simulink library "SaliencyLib"  (Simulink 7.1)
undefined symbols (not defined in the file): isc, IScale, isr, oa
libraries: SaliencyLib x77
settings Model: Creator=bruce  LastModifiedBy=bruce

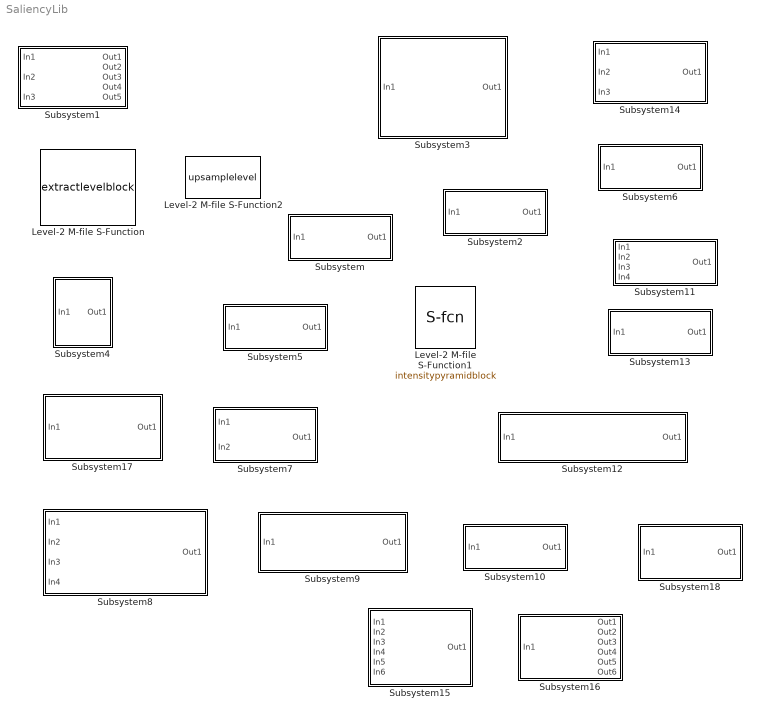
== system SaliencyLib ==
  Level-2 M-file S-Function : M-S-Function  FunctionName=extractlevelblock  Parameters=br,bc,pl,bo  mask(Extract Pyramid Level){br=332, bc=500, pl=2, bo=0}
      mask prompts: br "base rows:"; bc "base cols:"; pl "pyramid level:"; bo "base offset:"
      mask help:
      | Extracts one scale level from a multi-resolution pyramid
      | (that previously was packed into a matrix).
      mask Help:
      | For parameters are required.  Base rows and columns are the
      | dimensions of the level 0 image.  The pyramid level is the
      | resolution level that will be output. Base offset is normally
      | zero, but if the input pyramid was obtained by extracting
      | level n from a pyramid with level 0 dimensions given by the
      | base row and col parameter, then the base offset should be
      | set to n to give the correct input pyramid dimensions.
      mask Display: fprintf('EXTRACT\nLEVEL %s\n(%s x %s)', get_param(gcb, 'pl'),get_param(gcb,'br'),get_param(gcb,'bc'))
  Level-2 M-file S-Function1 : M-S-Function  FunctionName=intensitypyramidblock  Parameters=sr,sc,sl,bo  mask(Multi-Resolution Image Pyramid){sr=332, sc=500, sl=8, bo=0}
      mask prompts: sr "source rows:"; sc "source cols:"; sl "levels:"; bo "base offset:"
      mask help:
      | Constructs a multi-scale image pyramid from the input image
      | and outputs this pyramid packed into a 2-D matrix.
      mask Help:
      | Four parameters (sr,sc,sl,bo) are required.
      | 
      | sr and sc are the (nominal) row and column dimensions of the
      | input source image.
      | 
      | sl is the desired number of levels for the output pyramid.
      | 
      | bo is normally zero, but can be used to implicitly specify
      | the input image dimensions when the input is known to be
      | itself a level bo image from a pyramid derived from a base
      | image with dimensions sr by sc.
      mask Display: fprintf('PYRAMID\n(%s x %s)\n%s LEVEL', get_param(gcb,'sr'),get_param(gcb,'sc'),get_param(gcb,'sl'))
  Level-2 M-file S-Function2 : M-S-Function  FunctionName=upsamplelevel  Parameters=br,bc,fl,cl  mask(Upsample Image Pyramid Level){br=332, bc=500, fl=2, cl=5}
      mask prompts: br "base rows:"; bc "base cols:"; fl "fine level:"; cl "coarse level:"
      mask help:
      | Upsample a coarse resolution (higher) level image
      | to the resolution of a finer (lower) level image by simple
      | pixel replication.
      mask Help:
      | PARAMETERS:
      | base row, cols - level 0 image dimensions for the input pyramid.
      | fine level - the scale for the output image.
      | coarse level - the scale for the input image.
      mask Display: fprintf('UPSAMPLE\nLEVEL %s -> %s',get_param(gcb,'cl'),get_param(gcb,'fl'))
  Subsystem : Subsystem
      mask Type: Matrix Maximum
      mask Description: Outputs the value of the largest element in the input matrix.
      mask Display:
      | disp('MATRIX\nMAX')
      | port_label('input',1,'IMG')
      | port_label('output',1,'MAX')
  Subsystem1 : Subsystem  Tag=Color Map
      mask Type: Color Mapping
      mask Description:
      | Maps conventional RGB color component images to
      | intensity plus RGBY channels used by saliency algorithm.
      mask Display:
      | disp('COLOR\nMAPPING')
      | port_label('input',1,'r')
      | port_label('input',2','g')
      | port_label('input',3,'b')
      | port_label('output',1,'I')
      | port_label('output',2,'R')
      | port_label('output',3,'G')
      | port_label('output',4','B')
      | port_label('output',5,'Y')
  Subsystem10 : Subsystem  mask(Multi-Scale Color Opponent Saliency Channel){bRows=0, bCols=0}
      mask prompts: bRows "base rows:"; bCols "base cols:"
      mask help:
      | Outputs a bus containing color opponent saliency maps for
      | six different center-surround scale pairs.
      mask Display: fprintf('MULTI-SCALE\nCOLOR OPP\n(%s x %s)', get_param(gcb,'bRows'),get_param(gcb,'bCols'))
  Subsystem11 : Subsystem  mask(Color Based Saliency Channel){br=332, bc=500}
      mask prompts: br "base rows:"; bc "base cols:"
      mask help:
      | Outputs saliency map based on multi-scale double color
      | opponent center-surround differences in the input image.
      mask Display: fprintf('COLOR CHANNEL\n(%s x %s)',get_param(gcb,'br'),get_param(gcb,'bc'))
  Subsystem12 : Subsystem  mask(Single Orientation Saliency Channel){isr=332, isc=500, oa=0}
      mask prompts: isr "source rows:"; isc "source cols:"; oa "orientation angle:"
      mask help:
      | Outputs saliency map based on multi-scale center-surround
      | feature orientation differences for a single, parametrically
      | specified orientation.
      mask Display: fprintf('ORIENTED CHANNEL (%s DEG)\n(%s X %s)', get_param(gcb, 'oa'), get_param(gcb,'isr'),get_param(gcb,'isc'))
  Subsystem13 : Subsystem  mask(Multi-Orientation Based Saliency Channel){sr=0, sc=0}
      mask prompts: sr "source rows:"; sc "source cols:"
      mask help:
      | Outputs saliency map based on multi-scale, multi-orientation
      | center-surround feature orientation differences.
      mask Display: fprintf('MULTI-ORIENTED\nCHANNEL\n(%s x %s)',get_param(gcb,'sr'),get_param(gcb,'sc'))
  Subsystem14 : Subsystem  mask(Three Channel Saliency){inRows=332, inCols=500}
      mask prompts: inRows "input rows:"; inCols "input cols:"
      mask help:
      | Implements a three channel (intensity, orientation, color)
      | saliency map computaion based on the 1998 PAMI paper.
      mask Display:
      | fprintf('I-O-C CHANNEL\nSALIENCY\n(%s x %s)', get_param(gcb,'inRows'),get_param(gcb,'inCols'))
      | port_label('input',1,'r')
      | port_label('input',2,'g')
      | port_label('input',3,'b')
      | port_label('output',1,'SAL')
  Subsystem15 : Subsystem
      mask Type: Multi-Scale Image Bus Creator
      mask Description:
      | Provides a standardized means of assembling a multi-scale
      | collection of images into a bus.
      mask Display: disp('X-SCALE BUS\nCREATOR')
  Subsystem16 : Subsystem
      mask Type: Multi-Scale Image Bus Selector
      mask Description:
      | Provides a standardized connection to the bus created by
      | "X-SCALE BUS CREATOR" and un-packs bus components to separate
      | outputs.
      mask Display: disp('X-SCALE BUS\nSELECTOR')
  Subsystem17 : Subsystem  mask(Cross-Scale Summation){brxs=322, bcxs=500, L1off=0, L2off=0}
      mask prompts: brxs "base rows:"; bcxs "base cols:"; L1off "level one offset:"; L2off "level two offset:"
      mask help:
      | Output is the sum of six input center-surround absolute
      | difference maps at three different scales. Scales are
      | combined by downsampling.
      mask Display: fprintf('X-SCALE\nCOMBINE\n(%s x %s)\n%d-%d',get_param(gcb,'brxs'),get_param(gcb,'bcxs'),L1off,L2off)
  Subsystem18 : Subsystem  AncestorBlock=SaliencyLib/Subsystem12/Subsystem2  mask(Orientation Image Pyramid){sr=isr, sc=isc, pl=8, a=oa}
      mask prompts: sr "source rows:"; sc "source cols:"; pl "levels"; a "angle:"
      mask help:
      | Outputs a multi-scale pyramid obtained by applying a Gabor
      | kernel (with a parametrically specified orientation) to the
      | input image. The output pyramid is packed into a 2-D array.
      mask Display:
      | fprintf('ORIENT\nPYRAMID\n%s',get_param(gcb,'a'))
      | port_label('output',1,'PYR')
      | port_label('input',1,'IMG')
  Subsystem2 : Subsystem
      mask Type: Intensity Pyramid (DEPRECATED)
      mask Description:
      | Constructs a multi-scale image pyramid from the input matrix.
      | All of the pyramid levels are packed into a 2-D matrix.
      mask Display:
      | disp('INTENSITY\nPYRAMID')
      | port_label('output',1,'PYR')
      | port_label('input',1,'IMG')
  Subsystem3 : Subsystem  mask(Cross Level Difference){isr=0, isc=0}
      mask prompts: isr "input rows"; isc "input cols"
      mask help:
      | Computes absolute difference of scale 2 and 5 levels of an
      | image pyramid (upsampling the scale 5 image).
      mask Display:
      | port_label('input',1,'PYR')
      | port_label('output',1,'IMG')
      | fprintf('X-LEVEL DIFF\n(%d X %d)', isr, isc)
  Subsystem4 : Subsystem
      mask Type: Average of Local Maxima
      mask Description: Outputs average value of local maxima in the input image.
      mask Display: disp('AVG\nLOCAL\nMAX')
  Subsystem5 : Subsystem
      mask Type: Local Inhibition (Saliency Normalization)
      mask Description:
      | Scales input image based on difference of the global maximum
      | and the average of the local maxima.
      mask Display: disp('LOCAL\nINHIBIT')
  Subsystem6 : Subsystem  mask(Intensity Based Saliency Channel){isr=256, isc=256}
      mask prompts: isr "source rows:"; isc "source cols:"
      mask help:
      | Outputs a saliency map based on mulit-scale center-surround
      | intensity differences in the input image.
      mask Display: fprintf('INTENSITY CHANNEL\n(%s X %s)', get_param(gcb,'isr'),get_param(gcb,'isc'))
  Subsystem7 : Subsystem  mask(Color Opponent Pair Differences){br=332, bc=500, cl=2, sl=5}
      mask prompts: br "base rows:"; bc "base cols:"; cl "center level:"; sl "surround level:"
      mask help:
      | Computes multi-scale center-surround differences
      | for color opponent pairs.
      mask Display: fprintf('COLOR OPP\n(%s x %s)\n(%s -> %s)', get_param(gcb, 'br'), get_param(gcb, 'bc'), get_param(gcb, 'cl'), get_param(gcb, 'sl'))
  Subsystem8 : Subsystem  mask(Multi-Resolution Color Pyramid){br=332, bc=500}
      mask prompts: br "base rows:"; bc "base cols:"
      mask help:
      | Outputs a bus containing multi-resolution pyramids for each
      | of the four input color channel images.
      mask Display:
      | fprintf('COLOR PYRAMID\n(%s x %s)', get_param(gcb, 'br'), get_param(gcb, 'bc'))
      | port_label('input', 1, 'R')
      | port_label('input', 2', 'G')
      | port_label('input', 3, 'B')
      | port_label('input', 4, 'Y')
      | port_label('output', 1, 'CLRPY')
  Subsystem9 : Subsystem  mask(Single Resolution Color Opponent Saliency Channel){br=332, bc=500, cl=2, sl=5}
      mask prompts: br "base rows:"; bc "base cols:"; cl "center level:"; sl "surround level:"
      mask help:
      | Outputs a color opponent based saliency map for a
      | parametrically specified pair of center and surround
      | resolution scales.
      mask Display:
      | fprintf('CLR LEVEL\n(%s x %s)\n%s -> %s',get_param(gcb, 'br'),get_param(gcb, 'bc'),get_param(gcb,'cl'),get_param(gcb,'sl'))
      | port_label('input', 1, 'CLRPY')
      | port_label('output', 1, 'CPAIR')

== system SaliencyLib/Subsystem ==
  In1 : Inport  OutDataType=sfix(16)  OutScaling=2^0
  MATLAB Fcn : MATLABFcn  MATLABFcn=max(u(:))  Output1D=off
  Out1 : Outport  OutDataType=sfix(16)  OutScaling=2^0
  wires:
  MATLAB Fcn/1 -> Out1/1
  In1/1 -> MATLAB Fcn/1

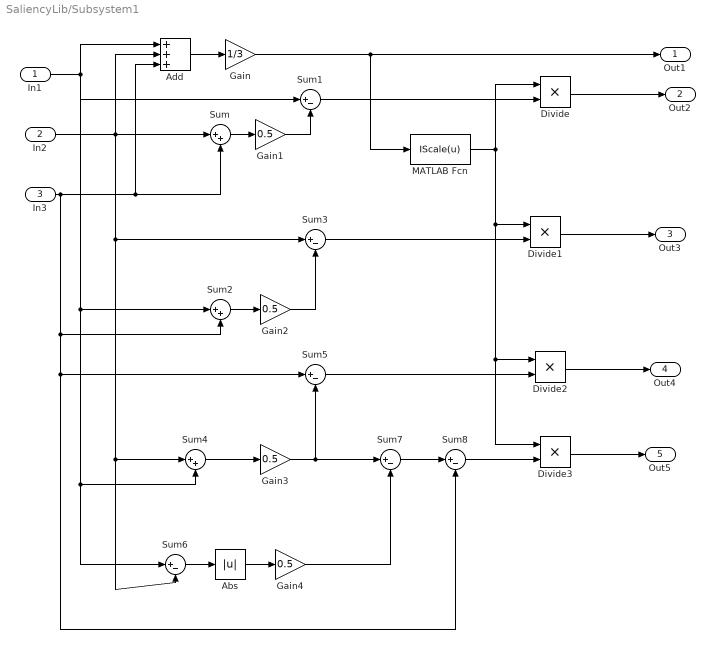
== system SaliencyLib/Subsystem1 ==
  In1 : Inport  OutDataType=sfix(16)  OutScaling=2^0
  In2 : Inport  Port=2  OutDataType=sfix(16)  OutScaling=2^0
  In3 : Inport  Port=3  OutDataType=sfix(16)  OutScaling=2^0
  Abs : Abs  OutDataType=sfix(16)  OutScaling=2^0
  Add : Sum  Inputs=+++  OutDataType=sfix(16)  OutScaling=2^-10
  Divide{,1..3} (4 alike) : Product  Inputs=**  OutDataType=sfix(16)  OutScaling=2^-10
  Gain : Gain  Gain=1/3  ParameterDataType=sfix(16)  ParameterScaling=2^0  OutDataType=sfix(16)  OutScaling=2^0
  Gain{1..4} (4 alike) : Gain  Gain=0.5  ParameterDataType=sfix(16)  ParameterScaling=2^0  OutDataType=sfix(16)  OutScaling=2^0
  MATLAB Fcn : MATLABFcn  MATLABFcn=IScale(u)  Output1D=off
  Sum : Sum  Inputs=|++  OutDataType=sfix(16)  OutScaling=2^0
  Sum{1,3,5..8} (6 alike) : Sum  Inputs=|+-  OutDataType=sfix(16)  OutScaling=2^0
  Sum2 : Sum  Inputs=|++  OutDataType=sfix(16)  OutScaling=2^0
  Sum4 : Sum  Inputs=|++  OutDataType=sfix(16)  OutScaling=2^0
  Out1 : Outport  OutDataType=sfix(16)  OutScaling=2^0
  Out2 : Outport  Port=2  OutDataType=sfix(16)  OutScaling=2^0
  Out3 : Outport  Port=3  OutDataType=sfix(16)  OutScaling=2^0
  Out4 : Outport  Port=4  OutDataType=sfix(16)  OutScaling=2^0
  Out5 : Outport  Port=5  OutDataType=sfix(16)  OutScaling=2^0
  wires:
  MATLAB Fcn/1 -> Divide3/1, Divide2/1, Divide1/1, Divide/1
  Divide3/1 -> Out5/1
  Sum8/1 -> Divide3/2
  Sum7/1 -> Sum8/1
  Gain4/1 -> Sum7/2
  Abs/1 -> Gain4/1
  Sum6/1 -> Abs/1
  Divide2/1 -> Out4/1
  Divide1/1 -> Out3/1
  Sum5/1 -> Divide2/2
  Sum3/1 -> Divide1/2
  Divide/1 -> Out2/1
  Sum1/1 -> Divide/2
  Sum4/1 -> Gain3/1
  Gain3/1 -> Sum7/1, Sum5/2
  Gain2/1 -> Sum3/2
  Sum2/1 -> Gain2/1
  Gain1/1 -> Sum1/2
  Sum/1 -> Gain1/1
  Add/1 -> Gain/1
  Gain/1 -> MATLAB Fcn/1, Out1/1
  In3/1 -> Sum8/2, Sum5/1, Sum2/2, Sum/2, Add/3
  In2/1 -> Sum6/2, Sum4/1, Sum3/1, Sum/1, Add/2
  In1/1 -> Sum6/1, Sum4/2, Sum2/1, Sum1/1, Add/1

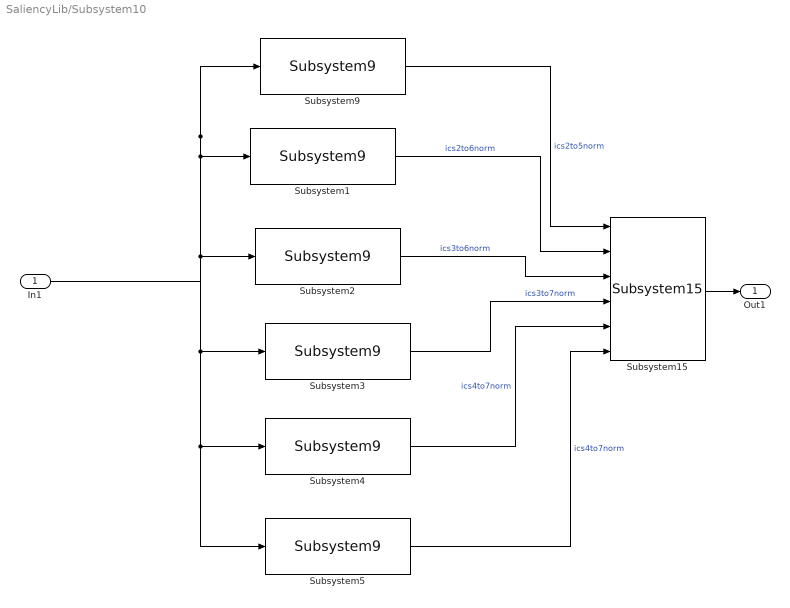
== system SaliencyLib/Subsystem10 ==
  In1 : Inport  OutDataType=sfix(16)  OutScaling=2^0
  Subsystem1 : SaliencyLib/Subsystem9  SystemSampleTime=-1  br=bRows  bc=bCols  cl=2  sl=6
  Subsystem15 : SaliencyLib/Subsystem15  SystemSampleTime=-1
  Subsystem2 : SaliencyLib/Subsystem9  SystemSampleTime=-1  br=bRows  bc=bCols  cl=3  sl=6
  Subsystem3 : SaliencyLib/Subsystem9  SystemSampleTime=-1  br=bRows  bc=bCols  cl=3  sl=7
  Subsystem4 : SaliencyLib/Subsystem9  SystemSampleTime=-1  br=bRows  bc=bCols  cl=4  sl=7
  Subsystem5 : SaliencyLib/Subsystem9  SystemSampleTime=-1  br=bRows  bc=bCols  cl=4  sl=8
  Subsystem9 : SaliencyLib/Subsystem9  SystemSampleTime=-1  br=bRows  bc=bCols  cl=2  sl=5
  Out1 : Outport  OutDataType=sfix(16)  OutScaling=2^0
  wires:
  In1/1 -> Subsystem9/1, Subsystem1/1, Subsystem2/1, Subsystem3/1, Subsystem4/1, Subsystem5/1
  Subsystem9/1 -> Subsystem15/1  "ics2to5norm"
  Subsystem1/1 -> Subsystem15/2  "ics2to6norm"
  Subsystem2/1 -> Subsystem15/3  "ics3to6norm"
  Subsystem3/1 -> Subsystem15/4  "ics3to7norm"
  Subsystem4/1 -> Subsystem15/5  "ics4to7norm"
  Subsystem5/1 -> Subsystem15/6  "ics4to7norm"
  Subsystem15/1 -> Out1/1

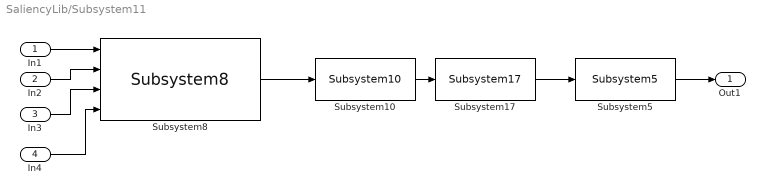
== system SaliencyLib/Subsystem11 ==
  In1 : Inport  OutDataType=sfix(16)  OutScaling=2^0
  In2 : Inport  Port=2  OutDataType=sfix(16)  OutScaling=2^0
  In3 : Inport  Port=3  OutDataType=sfix(16)  OutScaling=2^0
  In4 : Inport  Port=4  OutDataType=sfix(16)  OutScaling=2^0
  Subsystem10 : SaliencyLib/Subsystem10  SystemSampleTime=-1  bRows=br  bCols=bc
  Subsystem17 : SaliencyLib/Subsystem17  SystemSampleTime=-1  brxs=br  bcxs=bc  L1off=2  L2off=3
      link override Level-2 M-file S-Function6: bo=L2off
  Subsystem5 : SaliencyLib/Subsystem5  SystemSampleTime=-1
  Subsystem8 : SaliencyLib/Subsystem8  SystemSampleTime=-1  br=br  bc=bc
  Out1 : Outport  OutDataType=sfix(16)  OutScaling=2^0
  wires:
  In1/1 -> Subsystem8/1
  Subsystem8/1 -> Subsystem10/1
  Subsystem10/1 -> Subsystem17/1
  Subsystem17/1 -> Subsystem5/1
  Subsystem5/1 -> Out1/1
  In2/1 -> Subsystem8/2
  In3/1 -> Subsystem8/3
  In4/1 -> Subsystem8/4

== system SaliencyLib/Subsystem12 ==
  In1 : Inport  OutDataType=sfix(16)  OutScaling=2^0
  Subsystem12 : Subsystem
      mask Display: disp('NORMALIZE')
  Subsystem17 : SaliencyLib/Subsystem17  SystemSampleTime=-1  brxs=isr  bcxs=isc  L1off=2  L2off=3
  Subsystem2 : Subsystem  mask{sr=isr, sc=isc, pl=8, a=oa}
      mask prompts: sr "source rows:"; sc "source cols:"; pl "levels"; a "angle:"
      mask Display:
      | fprintf('ORIENT\nPYRAMID\n%s',get_param(gcb,'a'))
      | port_label('output',1,'PYR')
      | port_label('input',1,'IMG')
  Subsystem5 : SaliencyLib/Subsystem5  SystemSampleTime=-1
  Subsystem7 : Subsystem
      mask Display:
      | disp('C/S\nCOMBINE')
      | port_label('input',1,'PYR')
      | port_label('output',1,'I-BUS')
  Out1 : Outport  OutDataType=sfix(16)  OutScaling=2^0
  wires:
  In1/1 -> Subsystem2/1(In1)
  Subsystem2/1(Out1) -> Subsystem7/1(In1)
  Subsystem7/1(Out1) -> Subsystem12/1(In1)
  Subsystem17/1 -> Subsystem5/1
  Subsystem5/1 -> Out1/1
  Subsystem12/1(Out1) -> Subsystem17/1

== system SaliencyLib/Subsystem13 ==
  In1 : Inport  OutDataType=sfix(16)  OutScaling=2^0
  Add : Sum  Inputs=++++  OutDataType=sfix(16)  OutScaling=2^-10
  Subsystem1 : SaliencyLib/Subsystem12  SystemSampleTime=-1  isr=332  isc=500  oa=45
  Subsystem12 : SaliencyLib/Subsystem12  SystemSampleTime=-1  isr=332  isc=500  oa=0
  Subsystem2 : SaliencyLib/Subsystem12  SystemSampleTime=-1  isr=332  isc=500  oa=90
  Subsystem3 : SaliencyLib/Subsystem12  SystemSampleTime=-1  isr=332  isc=500  oa=135
  Subsystem5 : SaliencyLib/Subsystem5  SystemSampleTime=-1
  Out1 : Outport  OutDataType=sfix(16)  OutScaling=2^0
  wires:
  In1/1 -> Subsystem12/1, Subsystem1/1, Subsystem2/1, Subsystem3/1
  Subsystem12/1 -> Add/1
  Subsystem1/1 -> Add/2
  Subsystem2/1 -> Add/3
  Subsystem3/1 -> Add/4
  Add/1 -> Subsystem5/1
  Subsystem5/1 -> Out1/1

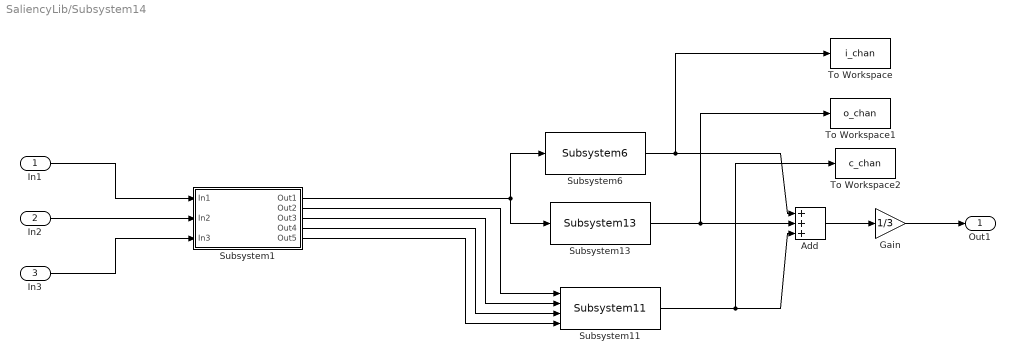
== system SaliencyLib/Subsystem14 ==
  In1 : Inport  OutDataType=sfix(16)  OutScaling=2^0
  In2 : Inport  Port=2  OutDataType=sfix(16)  OutScaling=2^0
  In3 : Inport  Port=3  OutDataType=sfix(16)  OutScaling=2^0
  Add : Sum  Inputs=+++  OutDataType=sfix(16)  OutScaling=2^-10
  Gain : Gain  Gain=1/3  ParameterDataType=sfix(16)  ParameterScaling=2^0  OutDataType=sfix(16)  OutScaling=2^0
  Subsystem1 : Subsystem
      mask Display:
      | disp('COLOR\nMAPPING')
      | port_label('input',1,'r')
      | port_label('input',2','g')
      | port_label('input',3,'b')
      | port_label('output',1,'I')
      | port_label('output',2,'R')
      | port_label('output',3,'G')
      | port_label('output',4','B')
      | port_label('output',5,'Y')
  Subsystem11 : SaliencyLib/Subsystem11  SystemSampleTime=-1  br=inRows  bc=inCols
  Subsystem13 : SaliencyLib/Subsystem13  SystemSampleTime=-1  sr=inRows  sc=inCols
  Subsystem6 : SaliencyLib/Subsystem6  SystemSampleTime=-1  isr=inRows  isc=inCols
      link override Subsystem17/Level-2 M-file S-Function: br=83  bc=125
      link override Subsystem17/Level-2 M-file S-Function1: sr=83  sc=125
      link override Subsystem17/Level-2 M-file S-Function2: sr=83  sc=125
      link override Subsystem17/Level-2 M-file S-Function3: sr=42  sc=63
      link override Subsystem17/Level-2 M-file S-Function4: sr=42  sc=63
      link override Subsystem17/Level-2 M-file S-Function5: br=83  bc=125
      link override Subsystem17/Level-2 M-file S-Function6: br=42  bc=63
      link override Subsystem17/Level-2 M-file S-Function7: br=42  bc=63
  To Workspace : ToWorkspace  VariableName=i_chan  SampleTime=-1  SaveFormat=Structure
  To Workspace1 : ToWorkspace  VariableName=o_chan  SampleTime=-1  SaveFormat=Structure
  To Workspace2 : ToWorkspace  VariableName=c_chan  SampleTime=-1  SaveFormat=Structure
  Out1 : Outport  OutDataType=sfix(16)  OutScaling=2^0
  wires:
  Add/1 -> Gain/1
  Gain/1 -> Out1/1
  Subsystem13/1 -> To Workspace1/1, Add/2
  Subsystem6/1 -> To Workspace/1, Add/1
  Subsystem11/1 -> To Workspace2/1, Add/3
  Subsystem1/5(Out5) -> Subsystem11/4
  Subsystem1/4(Out4) -> Subsystem11/3
  Subsystem1/3(Out3) -> Subsystem11/2
  Subsystem1/2(Out2) -> Subsystem11/1
  In3/1 -> Subsystem1/3(In3)
  In2/1 -> Subsystem1/2(In2)
  Subsystem1/1(Out1) -> Subsystem13/1, Subsystem6/1
  In1/1 -> Subsystem1/1(In1)

== system SaliencyLib/Subsystem15 ==
  In1 : Inport  OutDataType=sfix(16)  OutScaling=2^0
  In2 : Inport  Port=2  OutDataType=sfix(16)  OutScaling=2^0
  In3 : Inport  Port=3  OutDataType=sfix(16)  OutScaling=2^0
  In4 : Inport  Port=4  OutDataType=sfix(16)  OutScaling=2^0
  In5 : Inport  Port=5  OutDataType=sfix(16)  OutScaling=2^0
  In6 : Inport  Port=6  OutDataType=sfix(16)  OutScaling=2^0
  Bus Creator : BusCreator  Inputs='ics2to5norm','ics2to6norm','ics3to6norm','ics3to7norm','ics4to7norm','ics4to8norm'
  Out1 : Outport  OutDataType=sfix(16)  OutScaling=2^0
  wires:
  Bus Creator/1 -> Out1/1
  In1/1 -> Bus Creator/1  "ics2to5norm"
  In2/1 -> Bus Creator/2  "ics2to6norm"
  In3/1 -> Bus Creator/3  "ics3to6norm"
  In4/1 -> Bus Creator/4  "ics3to7norm"
  In5/1 -> Bus Creator/5  "ics4to7norm"
  In6/1 -> Bus Creator/6  "ics4to8norm"

== system SaliencyLib/Subsystem16 ==
  In1 : Inport  OutDataType=sfix(16)  OutScaling=2^0
  Bus Selector : BusSelector  OutputSignals=ics2to5norm,ics2to6norm,ics3to6norm,ics3to7norm,ics4to7norm,ics4to8norm
  Out1 : Outport  OutDataType=sfix(16)  OutScaling=2^0
  Out2 : Outport  Port=2  OutDataType=sfix(16)  OutScaling=2^0
  Out3 : Outport  Port=3  OutDataType=sfix(16)  OutScaling=2^0
  Out4 : Outport  Port=4  OutDataType=sfix(16)  OutScaling=2^0
  Out5 : Outport  Port=5  OutDataType=sfix(16)  OutScaling=2^0
  Out6 : Outport  Port=6  OutDataType=sfix(16)  OutScaling=2^0
  wires:
  In1/1 -> Bus Selector/1
  Bus Selector/1 -> Out1/1
  Bus Selector/2 -> Out2/1
  Bus Selector/3 -> Out3/1
  Bus Selector/4 -> Out4/1
  Bus Selector/5 -> Out5/1
  Bus Selector/6 -> Out6/1

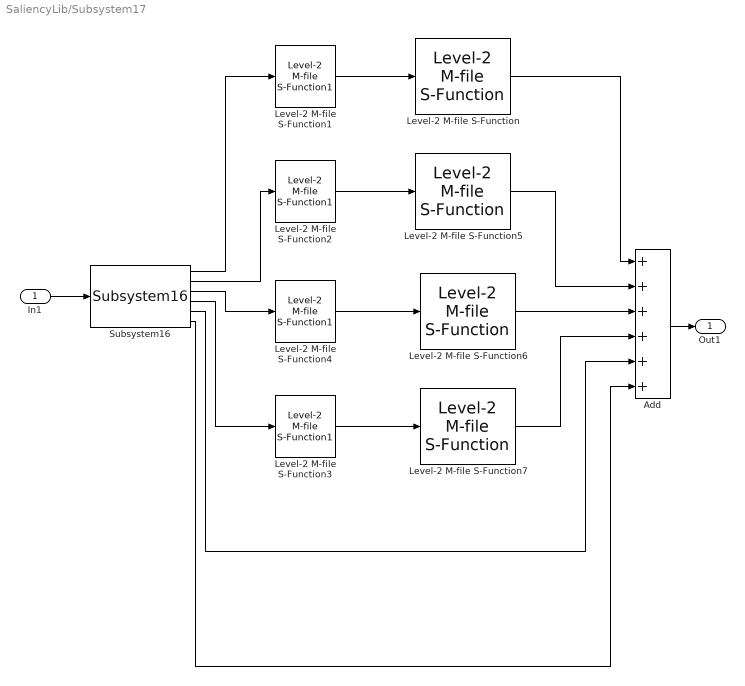
== system SaliencyLib/Subsystem17 ==
  In1 : Inport  OutDataType=sfix(16)  OutScaling=2^0
  Add : Sum  Inputs=++++++  OutDataType=sfix(16)  OutScaling=2^-10
  Level-2 M-file S-Function : SaliencyLib/Level-2 M-file S-Function  br=brxs  bc=bcxs  pl=2  bo=L1off
  Level-2 M-file S-Function1 : SaliencyLib/Level-2 M-file S-Function1  sr=brxs  sc=bcxs  sl=2  bo=0
  Level-2 M-file S-Function2 : SaliencyLib/Level-2 M-file S-Function1  sr=brxs  sc=bcxs  sl=2  bo=0
  Level-2 M-file S-Function3 : SaliencyLib/Level-2 M-file S-Function1  sr=brxs  sc=bcxs  sl=1  bo=0
  Level-2 M-file S-Function4 : SaliencyLib/Level-2 M-file S-Function1  sr=brxs  sc=bcxs  sl=1  bo=0
  Level-2 M-file S-Function5 : SaliencyLib/Level-2 M-file S-Function  br=brxs  bc=bcxs  pl=2  bo=L1off
  Level-2 M-file S-Function6 : SaliencyLib/Level-2 M-file S-Function  br=brxs  bc=bcxs  pl=1  bo=L2off
  Level-2 M-file S-Function7 : SaliencyLib/Level-2 M-file S-Function  br=brxs  bc=bcxs  pl=1  bo=L2off
  Subsystem16 : SaliencyLib/Subsystem16  SystemSampleTime=-1
  Out1 : Outport  OutDataType=sfix(16)  OutScaling=2^0
  wires:
  Add/1 -> Out1/1
  Level-2 M-file S-Function7/1 -> Add/4
  Level-2 M-file S-Function6/1 -> Add/3
  Level-2 M-file S-Function5/1 -> Add/2
  Level-2 M-file S-Function/1 -> Add/1
  Level-2 M-file S-Function3/1 -> Level-2 M-file S-Function7/1
  Level-2 M-file S-Function4/1 -> Level-2 M-file S-Function6/1
  Level-2 M-file S-Function2/1 -> Level-2 M-file S-Function5/1
  Level-2 M-file S-Function1/1 -> Level-2 M-file S-Function/1
  In1/1 -> Subsystem16/1
  Subsystem16/1 -> Level-2 M-file S-Function1/1
  Subsystem16/2 -> Level-2 M-file S-Function2/1
  Subsystem16/3 -> Level-2 M-file S-Function4/1
  Subsystem16/4 -> Level-2 M-file S-Function3/1
  Subsystem16/5 -> Add/5
  Subsystem16/6 -> Add/6

== system SaliencyLib/Subsystem18 ==
  In1 : Inport  OutDataType=sfix(16)  OutScaling=2^0
  Level-2 M-file S-Function : M-S-Function  FunctionName=orientationpyramidblock  Parameters=sr,sc,pl,a
  Out1 : Outport  OutDataType=sfix(16)  OutScaling=2^0
  wires:
  Level-2 M-file S-Function/1 -> Out1/1
  In1/1 -> Level-2 M-file S-Function/1

== system SaliencyLib/Subsystem2 ==
  In1 : Inport  OutDataType=sfix(16)  OutScaling=2^0
  MATLAB Fcn : MATLABFcn  MATLABFcn=IntensityPyramid  OutputDimensions=[499 500]  Output1D=off
  Out1 : Outport  OutDataType=sfix(16)  OutScaling=2^0
  wires:
  MATLAB Fcn/1 -> Out1/1
  In1/1 -> MATLAB Fcn/1

== system SaliencyLib/Subsystem3 ==
  In1 : Inport
  Abs : Abs  OutDataType=sfix(16)  OutScaling=2^0
  Level-2 M-file S-Function : SaliencyLib/Level-2 M-file S-Function  br=isr  bc=isc  pl=2  bo=0
  Level-2 M-file S-Function1 : SaliencyLib/Level-2 M-file S-Function  br=isr  bc=isc  pl=5  bo=0
  Level-2 M-file S-Function2 : SaliencyLib/Level-2 M-file S-Function2  br=isr  bc=isc  fl=2  cl=5
  Subtract : Sum  Inputs=+-  OutDataType=sfix(16)  OutScaling=2^-10
  Out1 : Outport
  wires:
  Level-2 M-file S-Function1/1 -> Level-2 M-file S-Function2/1
  Level-2 M-file S-Function2/1 -> Subtract/2
  Subtract/1 -> Abs/1
  Level-2 M-file S-Function/1 -> Subtract/1
  In1/1 -> Level-2 M-file S-Function1/1, Level-2 M-file S-Function/1
  Abs/1 -> Out1/1

== system SaliencyLib/Subsystem4 ==
  In1 : Inport  OutDataType=sfix(16)  OutScaling=2^0
  MATLAB Fcn1 : MATLABFcn  MATLABFcn=LocalMaxStats  Output1D=off
  Out1 : Outport  OutDataType=sfix(16)  OutScaling=2^0
  wires:
  In1/1 -> MATLAB Fcn1/1
  MATLAB Fcn1/1 -> Out1/1

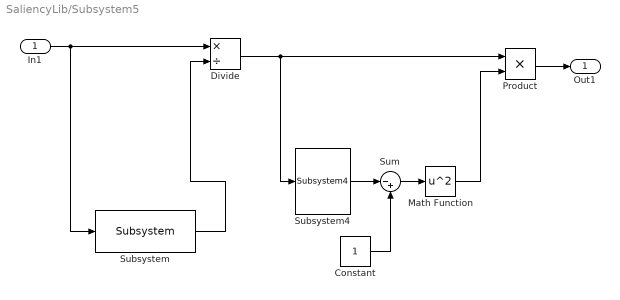
== system SaliencyLib/Subsystem5 ==
  In1 : Inport  OutDataType=sfix(16)  OutScaling=2^0
  Constant : Constant  OutDataType=sfix(16)  OutScaling=2^0
  Divide : Product  Inputs=*/  OutDataType=sfix(16)  OutScaling=2^-10
  Math Function : Math  Operator=square  OutDataType=sfix(16)  OutScaling=2^0  SaturateOnIntegerOverflow=on
  Product : Product  OutDataType=sfix(16)  OutScaling=2^0  RndMeth=Zero
  Subsystem : SaliencyLib/Subsystem  SystemSampleTime=-1
  Subsystem4 : SaliencyLib/Subsystem4  SystemSampleTime=-1
  Sum : Sum  Inputs=|-+  OutDataType=sfix(16)  OutScaling=2^0
  Out1 : Outport  OutDataType=sfix(16)  OutScaling=2^0
  wires:
  In1/1 -> Subsystem/1, Divide/1
  Subsystem/1 -> Divide/2
  Divide/1 -> Subsystem4/1, Product/1
  Constant/1 -> Sum/2
  Subsystem4/1 -> Sum/1
  Sum/1 -> Math Function/1
  Math Function/1 -> Product/2
  Product/1 -> Out1/1

== system SaliencyLib/Subsystem6 ==
  In1 : Inport  OutDataType=sfix(16)  OutScaling=2^0
  Level-2 M-file S-Function1 : SaliencyLib/Level-2 M-file S-Function1  sr=isr  sc=isc  sl=8  bo=0
  Subsystem12 : Subsystem
      mask Display: disp('NORMALIZE')
  Subsystem17 : SaliencyLib/Subsystem17  SystemSampleTime=-1  brxs=322  bcxs=500  L1off=0  L2off=0
  Subsystem5 : SaliencyLib/Subsystem5  SystemSampleTime=-1
  Subsystem7 : Subsystem
      mask Display:
      | disp('C/S\nCOMBINE')
      | port_label('input',1,'PYR')
      | port_label('output',1,'I-BUS')
  Out1 : Outport  OutDataType=sfix(16)  OutScaling=2^0
  wires:
  In1/1 -> Level-2 M-file S-Function1/1
  Level-2 M-file S-Function1/1 -> Subsystem7/1(In1)
  Subsystem7/1(Out1) -> Subsystem12/1(In1)
  Subsystem17/1 -> Subsystem5/1
  Subsystem5/1 -> Out1/1
  Subsystem12/1(Out1) -> Subsystem17/1

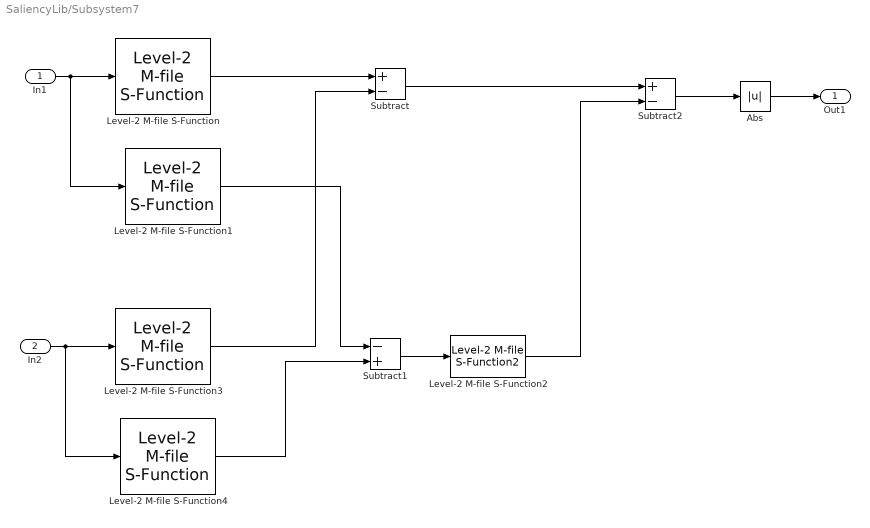
== system SaliencyLib/Subsystem7 ==
  In1 : Inport
  In2 : Inport  Port=2
  Abs : Abs  OutDataType=sfix(16)  OutScaling=2^0
  Level-2 M-file S-Function : SaliencyLib/Level-2 M-file S-Function  br=br  bc=bc  pl=cl  bo=0
  Level-2 M-file S-Function1 : SaliencyLib/Level-2 M-file S-Function  br=br  bc=bc  pl=sl  bo=0
  Level-2 M-file S-Function2 : SaliencyLib/Level-2 M-file S-Function2  br=br  bc=bc  fl=cl  cl=sl
  Level-2 M-file S-Function3 : SaliencyLib/Level-2 M-file S-Function  br=br  bc=bc  pl=cl  bo=0
  Level-2 M-file S-Function4 : SaliencyLib/Level-2 M-file S-Function  br=br  bc=bc  pl=sl  bo=0
  Subtract : Sum  Inputs=+-  OutDataType=sfix(16)  OutScaling=2^-10
  Subtract1 : Sum  Inputs=-+  OutDataType=sfix(16)  OutScaling=2^-10
  Subtract2 : Sum  Inputs=+-  OutDataType=sfix(16)  OutScaling=2^-10
  Out1 : Outport
  wires:
  Level-2 M-file S-Function/1 -> Subtract/1
  In1/1 -> Level-2 M-file S-Function1/1, Level-2 M-file S-Function/1
  Subtract1/1 -> Level-2 M-file S-Function2/1
  Level-2 M-file S-Function3/1 -> Subtract/2
  In2/1 -> Level-2 M-file S-Function3/1, Level-2 M-file S-Function4/1
  Level-2 M-file S-Function1/1 -> Subtract1/1
  Level-2 M-file S-Function4/1 -> Subtract1/2
  Abs/1 -> Out1/1
  Subtract/1 -> Subtract2/1
  Level-2 M-file S-Function2/1 -> Subtract2/2
  Subtract2/1 -> Abs/1

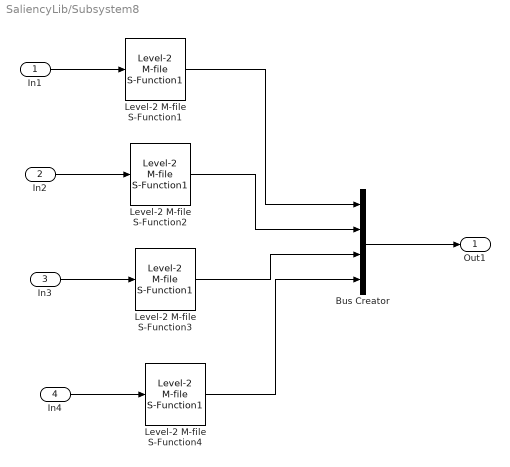
== system SaliencyLib/Subsystem8 ==
  In1 : Inport  OutDataType=sfix(16)  OutScaling=2^0
  In2 : Inport  Port=2  OutDataType=sfix(16)  OutScaling=2^0
  In3 : Inport  Port=3  OutDataType=sfix(16)  OutScaling=2^0
  In4 : Inport  Port=4  OutDataType=sfix(16)  OutScaling=2^0
  Bus Creator : BusCreator
  Level-2 M-file S-Function{1..4} (4 alike) : SaliencyLib/Level-2 M-file S-Function1  sr=332  sc=500  sl=8  bo=0
  Out1 : Outport  OutDataType=sfix(16)  OutScaling=2^0
  wires:
  In4/1 -> Level-2 M-file S-Function4/1
  In3/1 -> Level-2 M-file S-Function3/1
  In2/1 -> Level-2 M-file S-Function2/1
  In1/1 -> Level-2 M-file S-Function1/1
  Level-2 M-file S-Function1/1 -> Bus Creator/1
  Level-2 M-file S-Function2/1 -> Bus Creator/2
  Level-2 M-file S-Function3/1 -> Bus Creator/3
  Level-2 M-file S-Function4/1 -> Bus Creator/4
  Bus Creator/1 -> Out1/1

== system SaliencyLib/Subsystem9 ==
  In1 : Inport  OutDataType=sfix(16)  OutScaling=2^0
  Bus Selector : BusSelector  OutputSignals=signal1,signal2,signal3,signal4
  Subsystem1 : SaliencyLib/Subsystem7  SystemSampleTime=-1  br=br  bc=bc  cl=cl  sl=sl
  Subsystem2 : SaliencyLib/Subsystem5  SystemSampleTime=-1
  Subsystem5 : SaliencyLib/Subsystem5  SystemSampleTime=-1
  Subsystem7 : SaliencyLib/Subsystem7  SystemSampleTime=-1  br=br  bc=bc  cl=cl  sl=sl
  Sum : Sum  Inputs=|++  OutDataType=sfix(16)  OutScaling=2^0
  Out1 : Outport  OutDataType=sfix(16)  OutScaling=2^0
  wires:
  Sum/1 -> Out1/1
  In1/1 -> Bus Selector/1
  Bus Selector/1 -> Subsystem7/1  "<signal1>"
  Bus Selector/2 -> Subsystem7/2  "<signal2>"
  Bus Selector/3 -> Subsystem1/1  "<signal3>"
  Bus Selector/4 -> Subsystem1/2  "<signal4>"
  Subsystem7/1 -> Subsystem5/1
  Subsystem1/1 -> Subsystem2/1
  Subsystem5/1 -> Sum/1
  Subsystem2/1 -> Sum/2

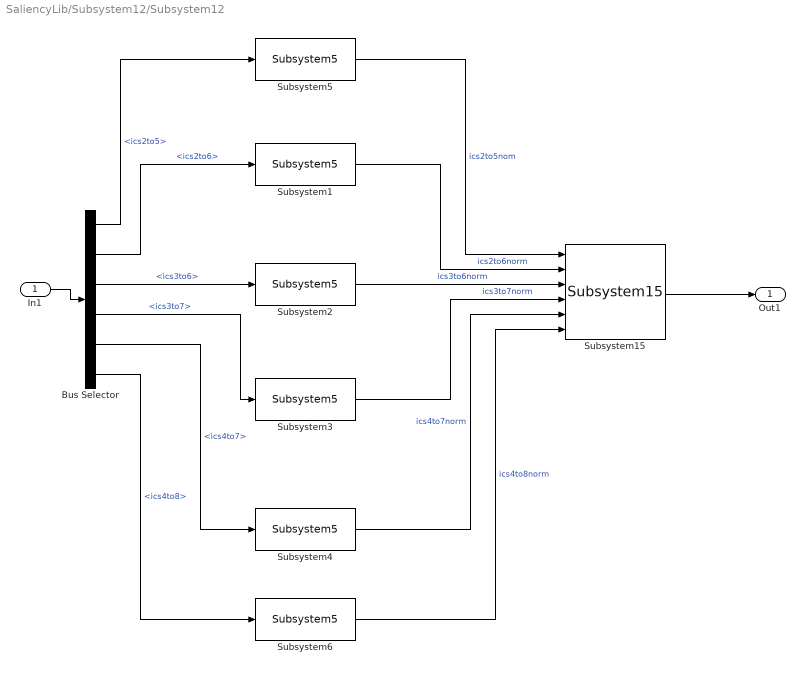
== system SaliencyLib/Subsystem12/Subsystem12 ==
  In1 : Inport  OutDataType=sfix(16)  OutScaling=2^0
  Bus Selector : BusSelector  OutputSignals=ics2to5,ics2to6,ics3to6,ics3to7,ics4to7,ics4to8
  Subsystem{1..6} (6 alike) : SaliencyLib/Subsystem5  SystemSampleTime=-1
  Subsystem15 : SaliencyLib/Subsystem15  SystemSampleTime=-1
  Out1 : Outport  OutDataType=sfix(16)  OutScaling=2^0
  wires:
  In1/1 -> Bus Selector/1
  Bus Selector/1 -> Subsystem5/1  "<ics2to5>"
  Bus Selector/2 -> Subsystem1/1  "<ics2to6>"
  Bus Selector/3 -> Subsystem2/1  "<ics3to6>"
  Bus Selector/4 -> Subsystem3/1  "<ics3to7>"
  Bus Selector/5 -> Subsystem4/1  "<ics4to7>"
  Bus Selector/6 -> Subsystem6/1  "<ics4to8>"
  Subsystem5/1 -> Subsystem15/1  "ics2to5nom"
  Subsystem1/1 -> Subsystem15/2  "ics2to6norm"
  Subsystem2/1 -> Subsystem15/3  "ics3to6norm"
  Subsystem3/1 -> Subsystem15/4  "ics3to7norm"
  Subsystem4/1 -> Subsystem15/5  "ics4to7norm"
  Subsystem6/1 -> Subsystem15/6  "ics4to8norm"
  Subsystem15/1 -> Out1/1

== system SaliencyLib/Subsystem12/Subsystem2 ==
  In1 : Inport  OutDataType=sfix(16)  OutScaling=2^0
  Level-2 M-file S-Function : M-S-Function  FunctionName=orientationpyramidblock  Parameters=sr,sc,pl,a
  Out1 : Outport  OutDataType=sfix(16)  OutScaling=2^0
  wires:
  In1/1 -> Level-2 M-file S-Function/1
  Level-2 M-file S-Function/1 -> Out1/1

== system SaliencyLib/Subsystem12/Subsystem7 ==
  In1 : Inport  OutDataType=sfix(16)  OutScaling=2^0
  Bus Creator : BusCreator  Inputs=6
  Subsystem1 : SaliencyLib/Subsystem3  SystemSampleTime=-1
      link override Level-2 M-file S-Function1: Parameters=332,500,6  pl=6
      link override Level-2 M-file S-Function2: cl=6
  Subsystem2 : SaliencyLib/Subsystem3  SystemSampleTime=-1
      link override Level-2 M-file S-Function: Parameters=332,500,3  pl=3
      link override Level-2 M-file S-Function1: Parameters=332,500,6  pl=6
      link override Level-2 M-file S-Function2: fl=3  cl=6
  Subsystem3 : SaliencyLib/Subsystem3  SystemSampleTime=-1
      link override Level-2 M-file S-Function: br=isr  bc=isc
      link override Level-2 M-file S-Function1: Parameters=332,500,5
  Subsystem4 : SaliencyLib/Subsystem3  SystemSampleTime=-1
      link override Level-2 M-file S-Function: Parameters=332,500,3  pl=3
      link override Level-2 M-file S-Function1: Parameters=332,500,7  pl=7
      link override Level-2 M-file S-Function2: fl=3  cl=7
  Subsystem5 : SaliencyLib/Subsystem3  SystemSampleTime=-1
      link override Level-2 M-file S-Function: Parameters=332,500,4  pl=4
      link override Level-2 M-file S-Function1: Parameters=332,500,7  pl=7
      link override Level-2 M-file S-Function2: fl=4  cl=7
  Subsystem6 : SaliencyLib/Subsystem3  SystemSampleTime=-1
      link override Level-2 M-file S-Function: Parameters=332,500,4  pl=4
      link override Level-2 M-file S-Function1: Parameters=332,500,8  pl=8
      link override Level-2 M-file S-Function2: fl=4  cl=8
  Out1 : Outport  OutDataType=sfix(16)  OutScaling=2^0
  wires:
  In1/1 -> Subsystem2/1, Subsystem4/1, Subsystem5/1, Subsystem6/1, Subsystem1/1, Subsystem3/1
  Subsystem1/1 -> Bus Creator/2  "ics2to6"
  Subsystem2/1 -> Bus Creator/3  "ics3to6"
  Subsystem3/1 -> Bus Creator/1  "ics2to5"
  Subsystem4/1 -> Bus Creator/4  "ics3to7"
  Bus Creator/1 -> Out1/1
  Subsystem5/1 -> Bus Creator/5  "ics4to7"
  Subsystem6/1 -> Bus Creator/6  "ics4to8"

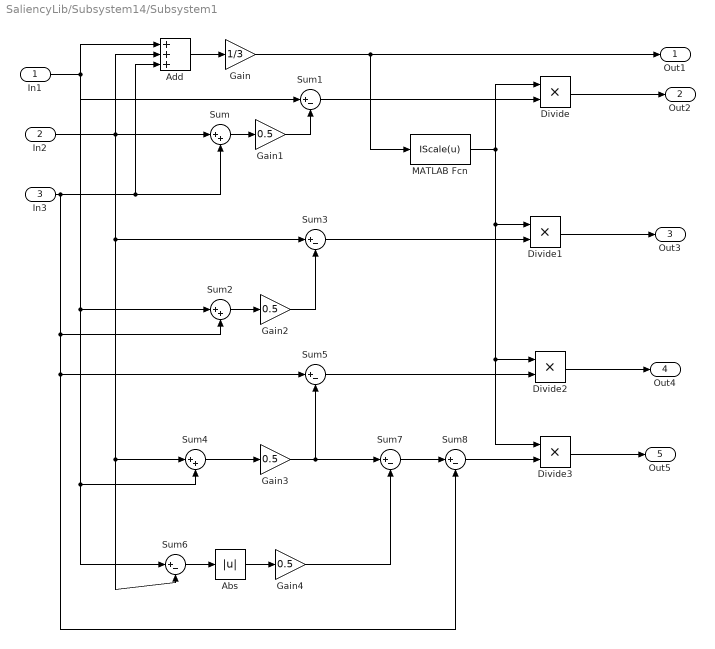
== system SaliencyLib/Subsystem14/Subsystem1 ==
  In1 : Inport  OutDataType=sfix(16)  OutScaling=2^0
  In2 : Inport  Port=2  OutDataType=sfix(16)  OutScaling=2^0
  In3 : Inport  Port=3  OutDataType=sfix(16)  OutScaling=2^0
  Abs : Abs  OutDataType=sfix(16)  OutScaling=2^0
  Add : Sum  Inputs=+++  OutDataType=sfix(16)  OutScaling=2^-10
  Divide{,1..3} (4 alike) : Product  Inputs=**  OutDataType=sfix(16)  OutScaling=2^-10
  Gain : Gain  Gain=1/3  ParameterDataType=sfix(16)  ParameterScaling=2^0  OutDataType=sfix(16)  OutScaling=2^0
  Gain{1..4} (4 alike) : Gain  Gain=0.5  ParameterDataType=sfix(16)  ParameterScaling=2^0  OutDataType=sfix(16)  OutScaling=2^0
  MATLAB Fcn : MATLABFcn  MATLABFcn=IScale(u)  Output1D=off
  Sum : Sum  Inputs=|++  OutDataType=sfix(16)  OutScaling=2^0
  Sum{1,3,5..8} (6 alike) : Sum  Inputs=|+-  OutDataType=sfix(16)  OutScaling=2^0
  Sum2 : Sum  Inputs=|++  OutDataType=sfix(16)  OutScaling=2^0
  Sum4 : Sum  Inputs=|++  OutDataType=sfix(16)  OutScaling=2^0
  Out1 : Outport  OutDataType=sfix(16)  OutScaling=2^0
  Out2 : Outport  Port=2  OutDataType=sfix(16)  OutScaling=2^0
  Out3 : Outport  Port=3  OutDataType=sfix(16)  OutScaling=2^0
  Out4 : Outport  Port=4  OutDataType=sfix(16)  OutScaling=2^0
  Out5 : Outport  Port=5  OutDataType=sfix(16)  OutScaling=2^0
  wires:
  In1/1 -> Add/1, Sum1/1, Sum2/1, Sum4/2, Sum6/1
  In2/1 -> Add/2, Sum/1, Sum3/1, Sum4/1, Sum6/2
  In3/1 -> Add/3, Sum/2, Sum2/2, Sum5/1, Sum8/2
  Gain/1 -> Out1/1, MATLAB Fcn/1
  Add/1 -> Gain/1
  Sum/1 -> Gain1/1
  Gain1/1 -> Sum1/2
  Sum2/1 -> Gain2/1
  Gain2/1 -> Sum3/2
  Gain3/1 -> Sum5/2, Sum7/1
  Sum4/1 -> Gain3/1
  Sum1/1 -> Divide/2
  Divide/1 -> Out2/1
  Sum3/1 -> Divide1/2
  Sum5/1 -> Divide2/2
  Divide1/1 -> Out3/1
  Divide2/1 -> Out4/1
  Sum6/1 -> Abs/1
  Abs/1 -> Gain4/1
  Gain4/1 -> Sum7/2
  Sum7/1 -> Sum8/1
  Sum8/1 -> Divide3/2
  Divide3/1 -> Out5/1
  MATLAB Fcn/1 -> Divide/1, Divide1/1, Divide2/1, Divide3/1

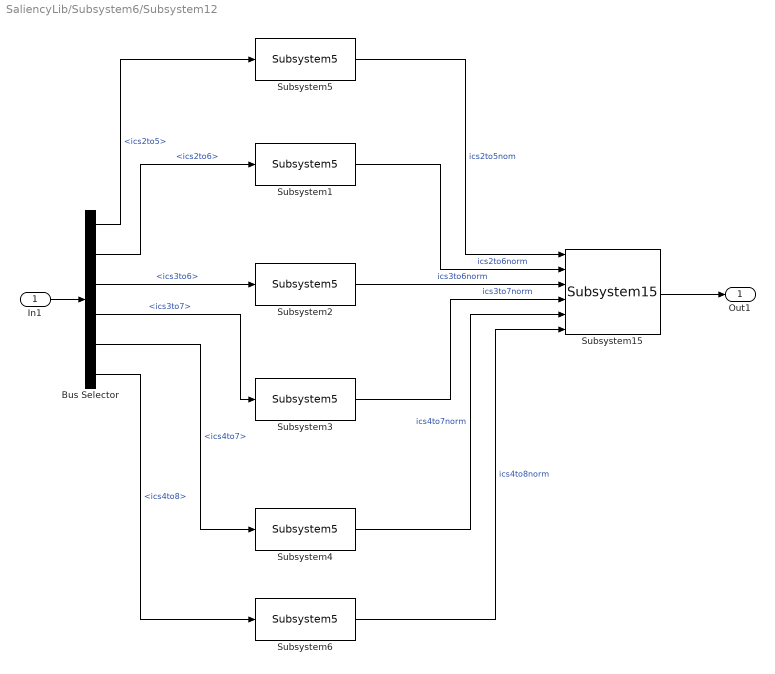
== system SaliencyLib/Subsystem6/Subsystem12 ==
  In1 : Inport  OutDataType=sfix(16)  OutScaling=2^0
  Bus Selector : BusSelector  OutputSignals=ics2to5,ics2to6,ics3to6,ics3to7,ics4to7,ics4to8
  Subsystem{1..6} (6 alike) : SaliencyLib/Subsystem5  SystemSampleTime=-1
  Subsystem15 : SaliencyLib/Subsystem15  SystemSampleTime=-1
  Out1 : Outport  OutDataType=sfix(16)  OutScaling=2^0
  wires:
  In1/1 -> Bus Selector/1
  Bus Selector/1 -> Subsystem5/1  "<ics2to5>"
  Bus Selector/2 -> Subsystem1/1  "<ics2to6>"
  Bus Selector/3 -> Subsystem2/1  "<ics3to6>"
  Bus Selector/4 -> Subsystem3/1  "<ics3to7>"
  Bus Selector/5 -> Subsystem4/1  "<ics4to7>"
  Bus Selector/6 -> Subsystem6/1  "<ics4to8>"
  Subsystem5/1 -> Subsystem15/1  "ics2to5nom"
  Subsystem1/1 -> Subsystem15/2  "ics2to6norm"
  Subsystem2/1 -> Subsystem15/3  "ics3to6norm"
  Subsystem3/1 -> Subsystem15/4  "ics3to7norm"
  Subsystem4/1 -> Subsystem15/5  "ics4to7norm"
  Subsystem6/1 -> Subsystem15/6  "ics4to8norm"
  Subsystem15/1 -> Out1/1

== system SaliencyLib/Subsystem6/Subsystem7 ==
  In1 : Inport  OutDataType=sfix(16)  OutScaling=2^0
  Bus Creator : BusCreator  Inputs=6
  Subsystem1 : SaliencyLib/Subsystem3  SystemSampleTime=-1  isr=isr  isc=isc
      link override Level-2 M-file S-Function1: Parameters=332,500,6  pl=6
      link override Level-2 M-file S-Function2: cl=6
  Subsystem2 : SaliencyLib/Subsystem3  SystemSampleTime=-1  isr=isr  isc=isc
      link override Level-2 M-file S-Function: Parameters=332,500,3  pl=3
      link override Level-2 M-file S-Function1: Parameters=332,500,6  pl=6
      link override Level-2 M-file S-Function2: fl=3  cl=6
  Subsystem3 : SaliencyLib/Subsystem3  SystemSampleTime=-1  isr=isr  isc=isc
      link override Level-2 M-file S-Function: br=isr  bc=isc
      link override Level-2 M-file S-Function1: Parameters=332,500,5
  Subsystem4 : SaliencyLib/Subsystem3  SystemSampleTime=-1  isr=isr  isc=isc
      link override Level-2 M-file S-Function: Parameters=332,500,3  pl=3
      link override Level-2 M-file S-Function1: Parameters=332,500,7  pl=7
      link override Level-2 M-file S-Function2: fl=3  cl=7
  Subsystem5 : SaliencyLib/Subsystem3  SystemSampleTime=-1  isr=isr  isc=isc
      link override Level-2 M-file S-Function: Parameters=332,500,4  pl=4
      link override Level-2 M-file S-Function1: Parameters=332,500,7  pl=7
      link override Level-2 M-file S-Function2: fl=4  cl=7
  Subsystem6 : SaliencyLib/Subsystem3  SystemSampleTime=-1  isr=isr  isc=isc
      link override Level-2 M-file S-Function: Parameters=332,500,4  pl=4
      link override Level-2 M-file S-Function1: Parameters=332,500,8  pl=8
      link override Level-2 M-file S-Function2: fl=4  cl=8
  Out1 : Outport  OutDataType=sfix(16)  OutScaling=2^0
  wires:
  In1/1 -> Subsystem2/1, Subsystem4/1, Subsystem5/1, Subsystem6/1, Subsystem1/1, Subsystem3/1
  Subsystem1/1 -> Bus Creator/2  "ics2to6"
  Subsystem2/1 -> Bus Creator/3  "ics3to6"
  Subsystem3/1 -> Bus Creator/1  "ics2to5"
  Subsystem4/1 -> Bus Creator/4  "ics3to7"
  Bus Creator/1 -> Out1/1
  Subsystem5/1 -> Bus Creator/5  "ics4to7"
  Subsystem6/1 -> Bus Creator/6  "ics4to8"
